simulink model "DrvStFtTrgtPosSelc"  (R2018b)
settings: Solver=FixedStepDiscrete  StartTime=0.0  StopTime=10.0  FixedStep=0.01  RelTol=1e-3
undefined symbols (not defined in the file or in its folder): KeSMSuSecRwStVIPFtrstRefAngle_Val, KeSMSw6sAcsEntryDrvStFtUpwdDnwdPos_Val, KeSMSw6sAcsEntryDrvStFtUpwdDnwdPosMax_Val, KeSMSw6sAcsEntryDrvStFtUpwdDnwdPosMin_Val, KeSMSw6sAcsExtDrvStFtUpwdDnwdPos_Val, KeSMSw6sAcsExtDrvStFtUpwdDnwdPosMax_Val, KeSMSw6sAcsExtDrvStFtUpwdDnwdPosMin_Val, KeSMSwAcsEntryDrvStFtUpwdDnwdPos_Val, KeSMSwAcsEntryDrvStFtUpwdDnwdPosMax_Val, KeSMSwAcsEntryDrvStFtUpwdDnwdPosMin_Val, KeSMSwAcsExtDrvStFtUpwdDnwdPos_Val, KeSMSwAcsExtDrvStFtUpwdDnwdPosMax_Val, KeSMSwAcsExtDrvStFtUpwdDnwdPosMin_Val
libraries: TrgtPosSelcLib x4
settings Model: ModifiedHistory=复位模式脚蹬由于没有外部标定，全都改为常量0  Creator=sn2xws  LastModifiedBy=sn2xws
settings DataIOCC: SaveFormat=StructureWithTime
settings OptimizationCC: DefaultParameterBehavior=Inlined  EnhancedBackFolding=on  PassReuseOutputArgsAs=Individual arguments  ZeroExternalMemoryAtStartup=off  ZeroInternalMemoryAtStartup=off  OptimizeBlockOrder=speed  DifferentSizesBufferReuse=on  OptimizationCustomize=off
settings DebuggingCC: ParameterTunabilityLossMsg=error
settings ModelReferenceCC: ModelReferenceNumInstancesAllowed=Single
settings SFSimCC: MATLABDynamicMemAlloc=off
settings RTWCC: SystemTargetFile=autosar.tlc  GenCodeOnly=on  TemplateMakefile=ert_default_tmf  Description=AUTOSAR  GenerateReport=on  IncludeHyperlinkInReport=on  LaunchReport=on  GenerateTraceInfo=on  GenerateTraceReport=on  GenerateTraceReportSl=on  GenerateTraceReportSf=on  GenerateTraceReportEml=on  GenerateCodeMetricsReport=on
settings CodeAppCC: ForceParamTrailComments=on  IgnoreCustomStorageClasses=off  OperatorAnnotations=on  SimulinkDataObjDesc=on  SFDataObjDesc=on  InsertBlockDesc=on
settings STFCustomTargetCC: TargetLangStandard=C99 (ISO)  MultiwordLength=256  ParMdlRefBuildCompliant=on  CompOptLevelCompliant=on  IncludeMdlTerminateFcn=off  CombineOutputUpdateFcns=on  SuppressErrorStatus=on  ERTCustomFileBanners=on  SupportNonFinite=off  SupportComplex=off  SupportContinuousTime=off  SupportNonInlinedSFcns=off  RemoveResetFunc=on  MATLABClassNameForMDSCustomization=Simulink.SoftwareTarget.ERTCustomization  AutosarCompliant=on  UseToolchainInfoCompliant=on  LookupTableObjectStructAxisOrder=2,1,3,4,...  LUTObjectStructOrderEvenSpacing=Size,Table,Breakpoints  SystemTargetFile=autosar.tlc
settings ERTTargetCC: TargetLangStandard=C99 (ISO)  ConcurrentExecutionCompliant=off  IncludeMdlTerminateFcn=off  SuppressErrorStatus=on  SupportNonFinite=off  SupportComplex=off  ModelStepFunctionPrototypeControlCompliant=off  CPPClassGenCompliant=off  AutosarCompliant=on  LookupTableObjectStructAxisOrder=2,1,3,4,...  LUTObjectStructOrderEvenSpacing=Size,Table,Breakpoints  InlinedParameterPlacement=NonHierarchical  ERTCustomFileTemplate=example_file_process.tlc  ERTFilePackagingFormat=Compact

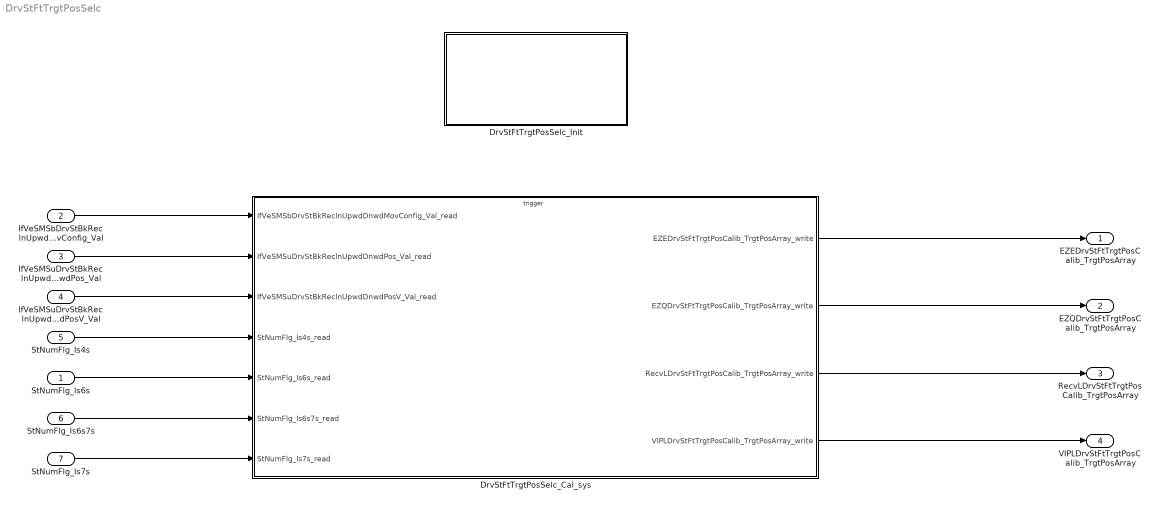
== system DrvStFtTrgtPosSelc ==
  StNumFlg_Is6s : Inport  OutDataTypeStr=boolean  PortDimensions=1
  IfVeSMSbDrvStBkReclnUpwdDnwdMovConfig_Val : Inport  Port=2  OutDataTypeStr=boolean  PortDimensions=1
  IfVeSMSuDrvStBkReclnUpwdDnwdPos_Val : Inport  Port=3  OutDataTypeStr=uint16  PortDimensions=1
  IfVeSMSuDrvStBkReclnUpwdDnwdPosV_Val : Inport  Port=4  OutDataTypeStr=boolean  PortDimensions=1
  StNumFlg_Is4s : Inport  Port=5  OutDataTypeStr=boolean  PortDimensions=1
  StNumFlg_Is6s7s : Inport  Port=6  OutDataTypeStr=boolean  PortDimensions=1
  StNumFlg_Is7s : Inport  Port=7  OutDataTypeStr=boolean  PortDimensions=1
  DrvStFtTrgtPosSelc_Cal_sys : Subsystem
  DrvStFtTrgtPosSelc_Init : Subsystem
  EZEDrvStFtTrgtPosCalib_TrgtPosArray : Outport  Description=|  OutDataTypeStr=uint16  PortDimensions=3
      | 0:Pos
      | 1:Max
      | 2:Min
  EZQDrvStFtTrgtPosCalib_TrgtPosArray : Outport  Description=|  Port=2  OutDataTypeStr=uint16  PortDimensions=3
      | 0:Pos
      | 1:Max
      | 2:Min
  RecvLDrvStFtTrgtPosCalib_TrgtPosArray : Outport  Description=|  Port=3  OutDataTypeStr=uint16  PortDimensions=3
      | 0:Pos
      | 1:Max
      | 2:Min
  VIPLDrvStFtTrgtPosCalib_TrgtPosArray : Outport  Description=|  Port=4  OutDataTypeStr=uint16  PortDimensions=3
      | 0:Pos
      | 1:Max
      | 2:Min
  wires:
  StNumFlg_Is6s/1 -> DrvStFtTrgtPosSelc_Cal_sys/5(StNumFlg_Is6s_read)
  IfVeSMSbDrvStBkReclnUpwdDnwdMovConfig_Val/1 -> DrvStFtTrgtPosSelc_Cal_sys/1(IfVeSMSbDrvStBkReclnUpwdDnwdMovConfig_Val_read)
  IfVeSMSuDrvStBkReclnUpwdDnwdPos_Val/1 -> DrvStFtTrgtPosSelc_Cal_sys/2(IfVeSMSuDrvStBkReclnUpwdDnwdPos_Val_read)
  IfVeSMSuDrvStBkReclnUpwdDnwdPosV_Val/1 -> DrvStFtTrgtPosSelc_Cal_sys/3(IfVeSMSuDrvStBkReclnUpwdDnwdPosV_Val_read)
  StNumFlg_Is4s/1 -> DrvStFtTrgtPosSelc_Cal_sys/4(StNumFlg_Is4s_read)
  StNumFlg_Is6s7s/1 -> DrvStFtTrgtPosSelc_Cal_sys/6(StNumFlg_Is6s7s_read)
  StNumFlg_Is7s/1 -> DrvStFtTrgtPosSelc_Cal_sys/7(StNumFlg_Is7s_read)
  DrvStFtTrgtPosSelc_Cal_sys/1(EZEDrvStFtTrgtPosCalib_TrgtPosArray_write) -> EZEDrvStFtTrgtPosCalib_TrgtPosArray/1
  DrvStFtTrgtPosSelc_Cal_sys/2(EZQDrvStFtTrgtPosCalib_TrgtPosArray_write) -> EZQDrvStFtTrgtPosCalib_TrgtPosArray/1
  DrvStFtTrgtPosSelc_Cal_sys/3(RecvLDrvStFtTrgtPosCalib_TrgtPosArray_write) -> RecvLDrvStFtTrgtPosCalib_TrgtPosArray/1
  DrvStFtTrgtPosSelc_Cal_sys/4(VIPLDrvStFtTrgtPosCalib_TrgtPosArray_write) -> VIPLDrvStFtTrgtPosCalib_TrgtPosArray/1

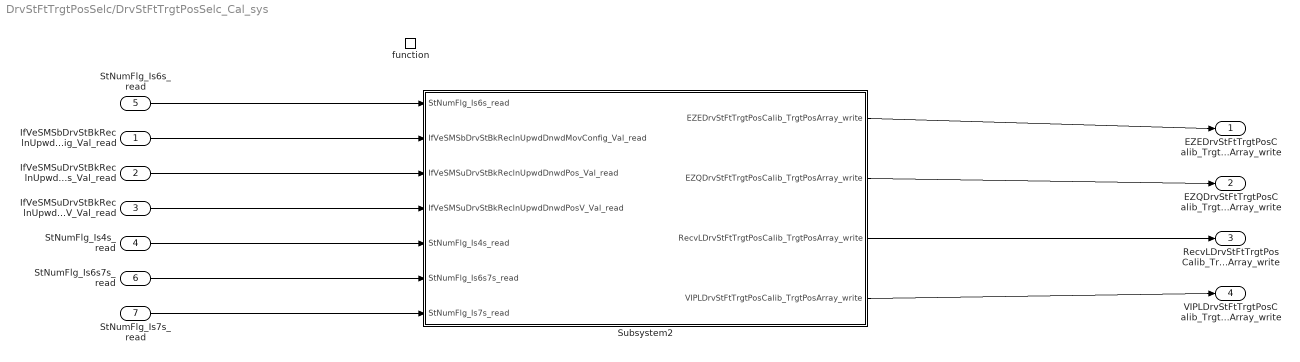
== system DrvStFtTrgtPosSelc/DrvStFtTrgtPosSelc_Cal_sys ==
  IfVeSMSbDrvStBkReclnUpwdDnwdMovConfig_Val_read : Inport
  IfVeSMSuDrvStBkReclnUpwdDnwdPos_Val_read : Inport  Port=2
  IfVeSMSuDrvStBkReclnUpwdDnwdPosV_Val_read : Inport  Port=3
  StNumFlg_Is4s_read : Inport  Port=4
  StNumFlg_Is6s_read : Inport  Port=5
  StNumFlg_Is6s7s_read : Inport  Port=6
  StNumFlg_Is7s_read : Inport  Port=7
  function : TriggerPort  TriggerType=function-call  IsSimulinkFunction=on  FunctionName=DrvStFtTrgtPosSelc_Cal  VariantControl=(inherit)
  Subsystem2 : Subsystem
  EZEDrvStFtTrgtPosCalib_TrgtPosArray_write : Outport
      settings: EnsureOutportIsVirtual=on
  EZQDrvStFtTrgtPosCalib_TrgtPosArray_write : Outport  Port=2
      settings: EnsureOutportIsVirtual=on
  RecvLDrvStFtTrgtPosCalib_TrgtPosArray_write : Outport  Port=3
      settings: EnsureOutportIsVirtual=on
  VIPLDrvStFtTrgtPosCalib_TrgtPosArray_write : Outport  Port=4
      settings: EnsureOutportIsVirtual=on
  wires:
  IfVeSMSbDrvStBkReclnUpwdDnwdMovConfig_Val_read/1 -> Subsystem2/2(IfVeSMSbDrvStBkReclnUpwdDnwdMovConfig_Val_read)
  IfVeSMSuDrvStBkReclnUpwdDnwdPos_Val_read/1 -> Subsystem2/3(IfVeSMSuDrvStBkReclnUpwdDnwdPos_Val_read)
  IfVeSMSuDrvStBkReclnUpwdDnwdPosV_Val_read/1 -> Subsystem2/4(IfVeSMSuDrvStBkReclnUpwdDnwdPosV_Val_read)
  StNumFlg_Is4s_read/1 -> Subsystem2/5(StNumFlg_Is4s_read)
  StNumFlg_Is6s_read/1 -> Subsystem2/1(StNumFlg_Is6s_read)
  StNumFlg_Is6s7s_read/1 -> Subsystem2/6(StNumFlg_Is6s7s_read)
  StNumFlg_Is7s_read/1 -> Subsystem2/7(StNumFlg_Is7s_read)
  Subsystem2/1(EZEDrvStFtTrgtPosCalib_TrgtPosArray_write) -> EZEDrvStFtTrgtPosCalib_TrgtPosArray_write/1
  Subsystem2/2(EZQDrvStFtTrgtPosCalib_TrgtPosArray_write) -> EZQDrvStFtTrgtPosCalib_TrgtPosArray_write/1
  Subsystem2/3(RecvLDrvStFtTrgtPosCalib_TrgtPosArray_write) -> RecvLDrvStFtTrgtPosCalib_TrgtPosArray_write/1
  Subsystem2/4(VIPLDrvStFtTrgtPosCalib_TrgtPosArray_write) -> VIPLDrvStFtTrgtPosCalib_TrgtPosArray_write/1

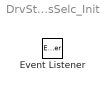
== system DrvStFtTrgtPosSelc/DrvStFtTrgtPosSelc_Init ==
  Event Listener : EventListener  EventName=reset

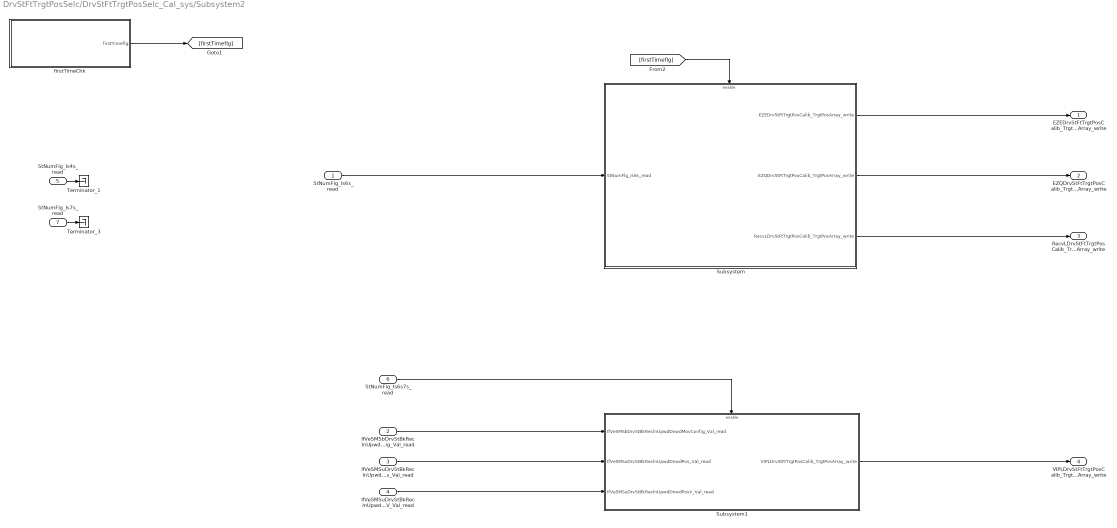
== system DrvStFtTrgtPosSelc/DrvStFtTrgtPosSelc_Cal_sys/Subsystem2 ==
  StNumFlg_Is6s_read : Inport
  IfVeSMSbDrvStBkReclnUpwdDnwdMovConfig_Val_read : Inport  Port=2
  IfVeSMSuDrvStBkReclnUpwdDnwdPos_Val_read : Inport  Port=3
  IfVeSMSuDrvStBkReclnUpwdDnwdPosV_Val_read : Inport  Port=4
  StNumFlg_Is4s_read : Inport  Port=5
  StNumFlg_Is6s7s_read : Inport  Port=6
  StNumFlg_Is7s_read : Inport  Port=7
  Subsystem : Subsystem
  Subsystem1 : Subsystem
  Terminator_1 : Terminator
  Terminator_3 : Terminator
  firstTimeChk : Stateflow chart  TreatAsAtomicUnit=on
  EZEDrvStFtTrgtPosCalib_TrgtPosArray_write : Outport
      settings: EnsureOutportIsVirtual=on
  EZQDrvStFtTrgtPosCalib_TrgtPosArray_write : Outport  Port=2
      settings: EnsureOutportIsVirtual=on
  RecvLDrvStFtTrgtPosCalib_TrgtPosArray_write : Outport  Port=3
      settings: EnsureOutportIsVirtual=on
  VIPLDrvStFtTrgtPosCalib_TrgtPosArray_write : Outport  Port=4
      settings: EnsureOutportIsVirtual=on
  wires:
  StNumFlg_Is6s_read/1 -> Subsystem/1(StNumFlg_Is6s_read)
  StNumFlg_Is7s_read/1 -> Terminator_3/1
  StNumFlg_Is4s_read/1 -> Terminator_1/1
  Subsystem/1(EZEDrvStFtTrgtPosCalib_TrgtPosArray_write) -> EZEDrvStFtTrgtPosCalib_TrgtPosArray_write/1
  firstTimeChk/1(firstTimeflg) -> [firstTimeflg]
  IfVeSMSbDrvStBkReclnUpwdDnwdMovConfig_Val_read/1 -> Subsystem1/1(IfVeSMSbDrvStBkReclnUpwdDnwdMovConfig_Val_read)
  Subsystem/2(EZQDrvStFtTrgtPosCalib_TrgtPosArray_write) -> EZQDrvStFtTrgtPosCalib_TrgtPosArray_write/1
  [firstTimeflg] -> Subsystem/Enable
  Subsystem1/1(VIPLDrvStFtTrgtPosCalib_TrgtPosArray_write) -> VIPLDrvStFtTrgtPosCalib_TrgtPosArray_write/1
  IfVeSMSuDrvStBkReclnUpwdDnwdPosV_Val_read/1 -> Subsystem1/3(IfVeSMSuDrvStBkReclnUpwdDnwdPosV_Val_read)
  Subsystem/3(RecvLDrvStFtTrgtPosCalib_TrgtPosArray_write) -> RecvLDrvStFtTrgtPosCalib_TrgtPosArray_write/1
  IfVeSMSuDrvStBkReclnUpwdDnwdPos_Val_read/1 -> Subsystem1/2(IfVeSMSuDrvStBkReclnUpwdDnwdPos_Val_read)
  StNumFlg_Is6s7s_read/1 -> Subsystem1/Enable

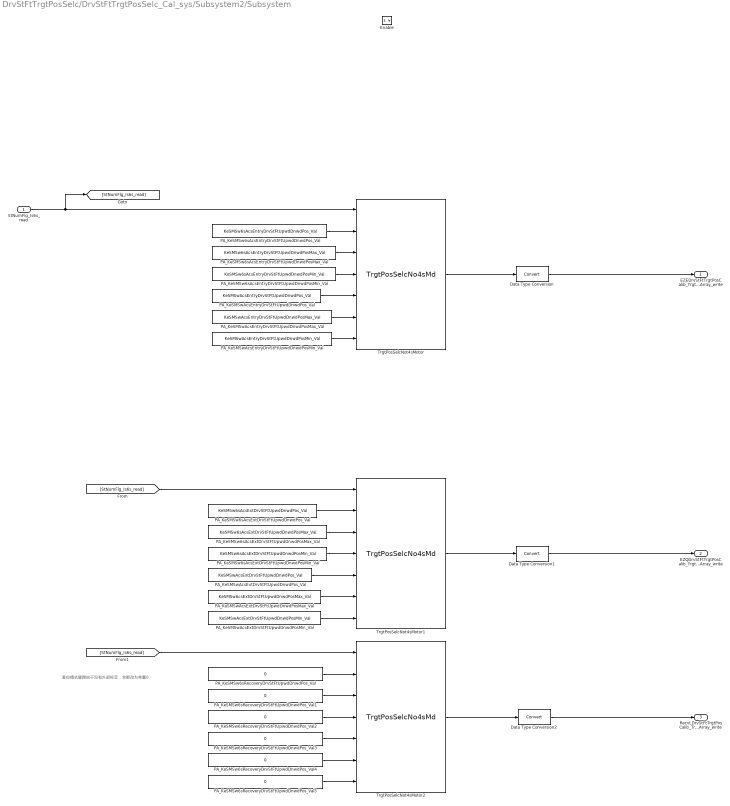
== system DrvStFtTrgtPosSelc/DrvStFtTrgtPosSelc_Cal_sys/Subsystem2/Subsystem ==
  note: 复位模式脚蹬由于没有外部标定，全都改为常量0
  StNumFlg_Is6s_read : Inport
  Enable : EnablePort
  Data Type Conversion : DataTypeConversion
  Data Type Conversion1 : DataTypeConversion
  Data Type Conversion2 : DataTypeConversion
  PA_KeSMSw6sAcsEntryDrvStFtUpwdDnwdPosMax_Val : Constant  Value=KeSMSw6sAcsEntryDrvStFtUpwdDnwdPosMax_Val
  PA_KeSMSw6sAcsEntryDrvStFtUpwdDnwdPosMin_Val : Constant  Value=KeSMSw6sAcsEntryDrvStFtUpwdDnwdPosMin_Val
  PA_KeSMSw6sAcsEntryDrvStFtUpwdDnwdPos_Val : Constant  Value=KeSMSw6sAcsEntryDrvStFtUpwdDnwdPos_Val
  PA_KeSMSw6sAcsExtDrvStFtUpwdDnwdPosMax_Val : Constant  Value=KeSMSw6sAcsExtDrvStFtUpwdDnwdPosMax_Val
  PA_KeSMSw6sAcsExtDrvStFtUpwdDnwdPosMin_Val : Constant  Value=KeSMSw6sAcsExtDrvStFtUpwdDnwdPosMin_Val
  PA_KeSMSw6sAcsExtDrvStFtUpwdDnwdPos_Val : Constant  Value=KeSMSw6sAcsExtDrvStFtUpwdDnwdPos_Val
  PA_KeSMSw6sRecoveryDrvStFtUpwdDnwdPos_Val{,1..5} (6 alike) : Constant  Value=0  OutDataTypeStr=uint16
  PA_KeSMSwAcsEntryDrvStFtUpwdDnwdPosMax_Val : Constant  Value=KeSMSwAcsEntryDrvStFtUpwdDnwdPosMax_Val
  PA_KeSMSwAcsEntryDrvStFtUpwdDnwdPosMin_Val : Constant  Value=KeSMSwAcsEntryDrvStFtUpwdDnwdPosMin_Val
  PA_KeSMSwAcsEntryDrvStFtUpwdDnwdPos_Val : Constant  Value=KeSMSwAcsEntryDrvStFtUpwdDnwdPos_Val
  PA_KeSMSwAcsExtDrvStFtUpwdDnwdPosMax_Val : Constant  Value=KeSMSwAcsExtDrvStFtUpwdDnwdPosMax_Val
  PA_KeSMSwAcsExtDrvStFtUpwdDnwdPosMin_Val : Constant  Value=KeSMSwAcsExtDrvStFtUpwdDnwdPosMin_Val
  PA_KeSMSwAcsExtDrvStFtUpwdDnwdPos_Val : Constant  Value=KeSMSwAcsExtDrvStFtUpwdDnwdPos_Val
  TrgtPosSelcNot4sMotor : TrgtPosSelcLib/TrgtPosSelcNo4sMd  SystemSampleTime=-1
  TrgtPosSelcNot4sMotor1 : TrgtPosSelcLib/TrgtPosSelcNo4sMd  SystemSampleTime=-1
  TrgtPosSelcNot4sMotor2 : TrgtPosSelcLib/TrgtPosSelcNo4sMd  SystemSampleTime=-1
  EZEDrvStFtTrgtPosCalib_TrgtPosArray_write : Outport
      settings: EnsureOutportIsVirtual=on
  EZQDrvStFtTrgtPosCalib_TrgtPosArray_write : Outport  Port=2
      settings: EnsureOutportIsVirtual=on
  RecvLDrvStFtTrgtPosCalib_TrgtPosArray_write : Outport  Port=3
      settings: EnsureOutportIsVirtual=on
  wires:
  PA_KeSMSwAcsExtDrvStFtUpwdDnwdPos_Val/1 -> TrgtPosSelcNot4sMotor1/5
  PA_KeSMSwAcsEntryDrvStFtUpwdDnwdPos_Val/1 -> TrgtPosSelcNot4sMotor/5
  TrgtPosSelcNot4sMotor/1 -> Data Type Conversion/1
  PA_KeSMSwAcsExtDrvStFtUpwdDnwdPosMax_Val/1 -> TrgtPosSelcNot4sMotor1/6
  PA_KeSMSw6sAcsEntryDrvStFtUpwdDnwdPosMax_Val/1 -> TrgtPosSelcNot4sMotor/3
  PA_KeSMSw6sRecoveryDrvStFtUpwdDnwdPos_Val4/1 -> TrgtPosSelcNot4sMotor2/6
  StNumFlg_Is6s_read/1 -> [StNumFlg_Is6s_read], TrgtPosSelcNot4sMotor/1
  PA_KeSMSwAcsEntryDrvStFtUpwdDnwdPosMin_Val/1 -> TrgtPosSelcNot4sMotor/7
  PA_KeSMSw6sAcsExtDrvStFtUpwdDnwdPosMin_Val/1 -> TrgtPosSelcNot4sMotor1/4
  PA_KeSMSw6sAcsExtDrvStFtUpwdDnwdPos_Val/1 -> TrgtPosSelcNot4sMotor1/2
  PA_KeSMSw6sAcsEntryDrvStFtUpwdDnwdPos_Val/1 -> TrgtPosSelcNot4sMotor/2
  [StNumFlg_Is6s_read] -> TrgtPosSelcNot4sMotor1/1
  TrgtPosSelcNot4sMotor1/1 -> Data Type Conversion1/1
  PA_KeSMSwAcsExtDrvStFtUpwdDnwdPosMin_Val/1 -> TrgtPosSelcNot4sMotor1/7
  TrgtPosSelcNot4sMotor2/1 -> Data Type Conversion2/1
  PA_KeSMSwAcsEntryDrvStFtUpwdDnwdPosMax_Val/1 -> TrgtPosSelcNot4sMotor/6
  PA_KeSMSw6sRecoveryDrvStFtUpwdDnwdPos_Val3/1 -> TrgtPosSelcNot4sMotor2/5
  PA_KeSMSw6sRecoveryDrvStFtUpwdDnwdPos_Val1/1 -> TrgtPosSelcNot4sMotor2/3
  PA_KeSMSw6sRecoveryDrvStFtUpwdDnwdPos_Val2/1 -> TrgtPosSelcNot4sMotor2/4
  PA_KeSMSw6sRecoveryDrvStFtUpwdDnwdPos_Val/1 -> TrgtPosSelcNot4sMotor2/2
  [StNumFlg_Is6s_read] -> TrgtPosSelcNot4sMotor2/1
  PA_KeSMSw6sRecoveryDrvStFtUpwdDnwdPos_Val5/1 -> TrgtPosSelcNot4sMotor2/7
  PA_KeSMSw6sAcsEntryDrvStFtUpwdDnwdPosMin_Val/1 -> TrgtPosSelcNot4sMotor/4
  PA_KeSMSw6sAcsExtDrvStFtUpwdDnwdPosMax_Val/1 -> TrgtPosSelcNot4sMotor1/3
  Data Type Conversion/1 -> EZEDrvStFtTrgtPosCalib_TrgtPosArray_write/1
  Data Type Conversion1/1 -> EZQDrvStFtTrgtPosCalib_TrgtPosArray_write/1
  Data Type Conversion2/1 -> RecvLDrvStFtTrgtPosCalib_TrgtPosArray_write/1

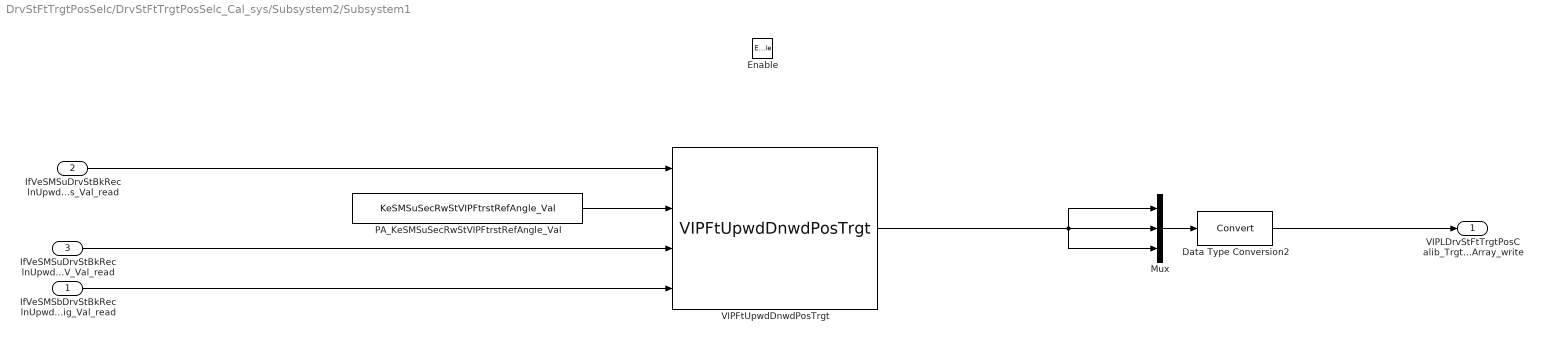
== system DrvStFtTrgtPosSelc/DrvStFtTrgtPosSelc_Cal_sys/Subsystem2/Subsystem1 ==
  IfVeSMSbDrvStBkReclnUpwdDnwdMovConfig_Val_read : Inport
  IfVeSMSuDrvStBkReclnUpwdDnwdPos_Val_read : Inport  Port=2
  IfVeSMSuDrvStBkReclnUpwdDnwdPosV_Val_read : Inport  Port=3
  Enable : EnablePort
  Data Type Conversion2 : DataTypeConversion
  Mux : Mux  Inputs=3
  PA_KeSMSuSecRwStVIPFtrstRefAngle_Val : Constant  Value=KeSMSuSecRwStVIPFtrstRefAngle_Val
  VIPFtUpwdDnwdPosTrgt : TrgtPosSelcLib/VIPFtUpwdDnwdPosTrgt  SystemSampleTime=-1
  VIPLDrvStFtTrgtPosCalib_TrgtPosArray_write : Outport  InitialOutput=0
  wires:
  VIPFtUpwdDnwdPosTrgt/1 -> Mux/3, Mux/1, Mux/2
  IfVeSMSuDrvStBkReclnUpwdDnwdPosV_Val_read/1 -> VIPFtUpwdDnwdPosTrgt/3
  PA_KeSMSuSecRwStVIPFtrstRefAngle_Val/1 -> VIPFtUpwdDnwdPosTrgt/2
  IfVeSMSbDrvStBkReclnUpwdDnwdMovConfig_Val_read/1 -> VIPFtUpwdDnwdPosTrgt/4
  IfVeSMSuDrvStBkReclnUpwdDnwdPos_Val_read/1 -> VIPFtUpwdDnwdPosTrgt/1
  Mux/1 -> Data Type Conversion2/1
  Data Type Conversion2/1 -> VIPLDrvStFtTrgtPosCalib_TrgtPosArray_write/1

== stateflow chart DrvStFtTrgtPosSelc/DrvStFtTrgtPosSelc_Cal_sys/Subsystem2/firstTimeChk ==
  (default) -> (junction 1)
  (junction 1) -> (junction 5) [order 1] : [chkflg ==0]
  (junction 1) -> (junction 3) [order 2] : {firstTimeflg = 0;}
  (junction 5) -> (junction 7) : {firstTimeflg = 1;
      | chkflg=1;}
  (junction 7) -> (junction 3)
  (junction 3) -> (junction 10)
  data: chkflg local boolean size=1; firstTimeflg output boolean size=1
